simulink model "bintang_transfer_function_02_Oktober"  (R2023a)
settings: Solver=VariableStepAuto  StartTime=0.0  StopTime=10.0  RelTol=1e-3
settings Model: Creator=Lenovo  LastModifiedBy=Lenovo

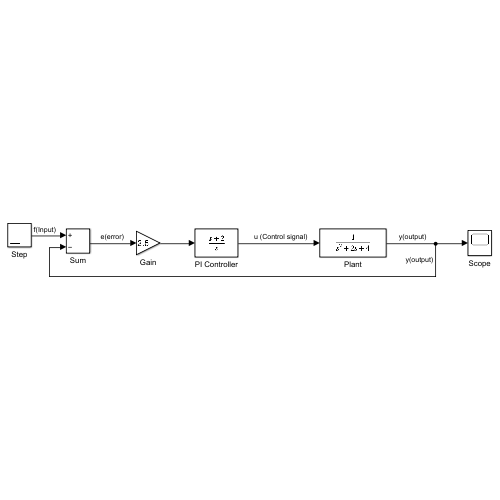
[thumbnail: Simulink's stored preview of the top-level diagram]
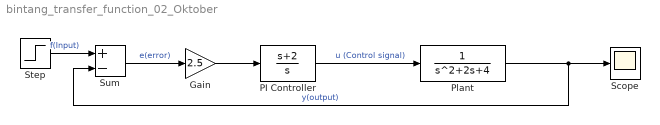
== system bintang_transfer_function_02_Oktober ==
  Gain : Gain  Gain=2.5
  PI Controller : TransferFcn  Numerator=[1 2]  Denominator=[1 0]
  Plant : TransferFcn  Denominator=[1 2 4]
  Scope : Scope
  Step : Step  After=0.5  SampleTime=0
  Sum : Sum  Inputs=+-
  wires:
  Plant/1 -> Sum/2, Scope/1  "y(output)"
  PI Controller/1 -> Plant/1  "u (Control signal)"
  Gain/1 -> PI Controller/1
  Sum/1 -> Gain/1  "e(error)"
  Step/1 -> Sum/1  "f(Input)"
